simulink model "power_sens"  (Simulink 6.6)
settings: Solver=ode45  StartTime=0.0  StopTime=10.0  RelTol=1e-3
settings Model: Creator=cmcrae  LastModifiedBy=cmcrae

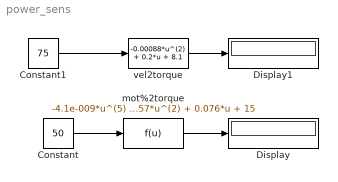
== system power_sens ==
  Constant : Constant  Value=50
  Constant1 : Constant  Value=75
  Display : Display
  Display1 : Display
  mot%2torque : Fcn  Expr=-4.1e-009*u^(5) + 6e-008*u^(4) + 5.8e-005*u^(3) - 0.0057*u^(2) + 0.076*u + 15
  vel2torque : Fcn  Expr=-0.00088*u^(2) + 0.2*u + 8.1
  wires:
  mot%2torque/1 -> Display/1
  Constant/1 -> mot%2torque/1
  Constant1/1 -> vel2torque/1
  vel2torque/1 -> Display1/1
